simulink model "sfcndemo_frame"  (Simulink 7.6)
settings: Solver=FixedStepDiscrete  SolverMode=SingleTasking  StartTime=0.0  StopTime=1  RelTol=1e-3
PreLoadFcn:
  | a=ones(1,256);a(96:110)=zeros(1,15);a(148:162)=zeros(1,15);a=[a', a'];
Description:
  | (Requires Signal Processing Blockset) Frame-Based Processing for Removing Sinusoidal Noise Using C-MEX S-functions
settings Model: Creator=The MathWorks Inc.  ExtModeAutoUpdateStatusClock=off
settings OptimizationCC: BlockReduction=off  BooleanDataType=off  InitFltsAndDblsToZero=on
settings DebuggingCC: SaveWithParameterizedLinksMsg=none  SignalResolutionControl=TryResolveAllWithWarning  SolverPrmCheckMsg=none  MultiTaskDSMMsg=warning  MultiTaskCondExecSysMsg=none
settings HardwareCC: TargetUnknown=on
settings RTWCC: RetainRTWFile=on  IncludeERTFirstTime=on
settings CodeAppCC: CustomSymbolStrFcn=$F$N$M
settings GRTTargetCC: TargetFcnLib=ansi_tfl_tmw.mat

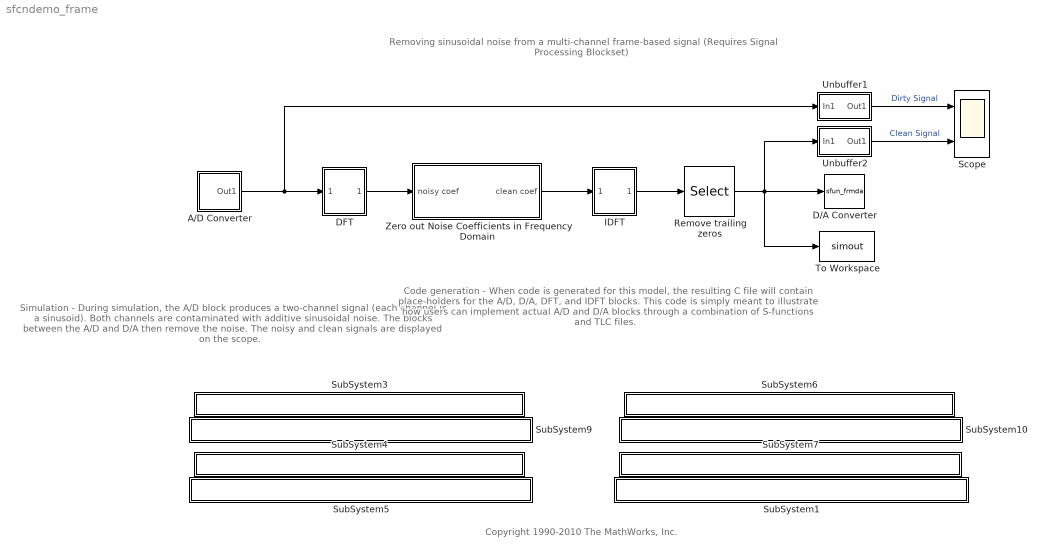
== system sfcndemo_frame ==
  note: Removing sinusoidal noise from a multi-channel frame-based signal
      | (Requires Signal Processing Blockset)
  note: Simulation -
      | During simulation, the A/D block produces
      | a two-channel signal (each channel is a sinusoid).
      | Both channels are contaminated with additive
      | sinusoidal noise. The blocks between the A/D and D/A
      | then remove the noise. The noisy and clean signals are
      | displayed on the scope.
  note: Code generation -
      | When code is generated for this model, the resulting C file
      | will contain place-holders for the A/D, D/A, DFT, and IDFT blocks.
      | This code is simply meant to illustrate how users can implement
      | actual A/D and D/A blocks through a combination of S-functions and
      | TLC files.
  note: Copyright 1990-2010 The MathWorks, Inc.
  A/D Converter : Subsystem  mask(A/D Converter){wf=Sine, amp=[10 5], freq=[5 10], Ts=0.005, fs=64, namp=4, nfreq=80}
      mask prompts: wf "Waveform for simulation"; amp "Amplitudes"; freq "Frequencies"; Ts "Sample time"; fs "Frame size"; namp "Noise amplitude for simulation"; nfreq "Noise frequency for simulation"
      mask help: During simulation, produces a constant or sinusoidal frame-based signal with additive sinusoidal noise. Multi-channel sinusoidal signals can be produced by giving a vector of frequncies or amplitudes. The same noise is added to all channels.
      mask StyleString: popup(Constant | Sine),edit,edit,edit,edit,edit,edit
      mask Display: disp('A/D')
  D/A Converter : S-Function  FunctionName=sfun_frmda  EnableBusSupport=off
      mask Type: D/A Converter
      mask Description: Frame-based D/A converter. Has no function during simulation.
      mask Display: disp('D/A')
  DFT : Subsystem  mask(DFT){ds=256}
      mask prompts: ds "DFT size"
      mask help: Compue the Discrete Fourer Transform
      mask Display: disp('DFT')
  IDFT : Subsystem
      mask Type: IDFT
      mask Description: Compute the inverse Discrete Fourier Transform.
      mask Display: disp('IDFT')
  Remove trailing zeros : Selector  NumberOfDimensions=2  IndexOptions=Index vector (dialog),Select all  Indices=1:64,-1  OutputSizes=1
  Scope : Scope  NumInputPorts=2
      settings: TimeRange=1  YMin=-12~-12  YMax=12~12
  SubSystem1 : Subsystem  mask{filename=sfun_frmunbuff.tlc}
      mask init:
      | x=sfundemo_maskdisp;
      settings: AttributesFormatString=\n  OpenFcn=sfundemo_openfcn
      mask Display: disp(x);
  SubSystem10 : Subsystem  mask{filename=sfun_frmdft.tlc}
      mask init:
      | x=sfundemo_maskdisp;
      settings: AttributesFormatString=\n  OpenFcn=sfundemo_openfcn
      mask Display: disp(x);
  SubSystem3 : Subsystem  mask{filename=sfun_frmad.c}
      mask init:
      | x=sfundemo_maskdisp;
      settings: AttributesFormatString=\n  OpenFcn=sfundemo_openfcn
      mask Display: disp(x);
  SubSystem4 : Subsystem  mask{filename=sfun_frmda.c}
      mask init:
      | x=sfundemo_maskdisp;
      settings: AttributesFormatString=\n  OpenFcn=sfundemo_openfcn
      mask Display: disp(x);
  SubSystem5 : Subsystem  mask{filename=sfun_frmda.tlc}
      mask init:
      | x=sfundemo_maskdisp;
      settings: AttributesFormatString=\n  OpenFcn=sfundemo_openfcn
      mask Display: disp(x);
  SubSystem6 : Subsystem  mask{filename=sfun_frmdft.c}
      mask init:
      | x=sfundemo_maskdisp;
      settings: AttributesFormatString=\n  OpenFcn=sfundemo_openfcn
      mask Display: disp(x);
  SubSystem7 : Subsystem  mask{filename=sfun_frmunbuff.c}
      mask init:
      | x=sfundemo_maskdisp;
      settings: AttributesFormatString=\n  OpenFcn=sfundemo_openfcn
      mask Display: disp(x);
  SubSystem9 : Subsystem  mask{filename=sfun_frmad.tlc}
      mask init:
      | x=sfundemo_maskdisp;
      settings: AttributesFormatString=\n  OpenFcn=sfundemo_openfcn
      mask Display: disp(x);
  To Workspace : ToWorkspace  VariableName=simout  SampleTime=-1  SaveFormat=Array
  Unbuffer1 : Subsystem
      mask Type: Frame Unbuffer
      mask Description: Unbuffer a frame-based signal
      mask Display: disp('Unbuffer')
  Unbuffer2 : Subsystem
      mask Type: Frame Unbuffer
      mask Description: Unbuffer a frame-based signal
      mask Display: disp('Unbuffer')
  Zero out Noise Coefficients in Frequency Domain : Subsystem
  wires:
  A/D Converter/1(Out1) -> DFT/1(In1), Unbuffer1/1(In1)
  DFT/1(Out1) -> Zero out Noise Coefficients in Frequency Domain/1(noisy coef)
  IDFT/1(Out1) -> Remove trailing zeros/1
  Remove trailing zeros/1 -> D/A Converter/1, Unbuffer2/1(In1), To Workspace/1
  Zero out Noise Coefficients in Frequency Domain/1(clean coef) -> IDFT/1(In1)
  Unbuffer2/1(Out1) -> Scope/2  "Clean Signal"
  Unbuffer1/1(Out1) -> Scope/1  "Dirty Signal"

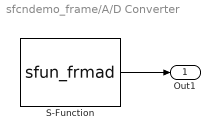
== system sfcndemo_frame/A/D Converter ==
  S-Function : S-Function  FunctionName=sfun_frmad  Parameters=wf,amp,freq,Ts,fs,namp,nfreq  SFunctionModules=sfun_frmad_wrapper  EnableBusSupport=off
  Out1 : Outport
  wires:
  S-Function/1 -> Out1/1

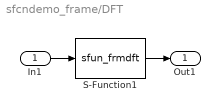
== system sfcndemo_frame/DFT ==
  In1 : Inport
  S-Function1 : S-Function  FunctionName=sfun_frmdft  Parameters=1,ds  SFunctionModules=sfun_frmdft_wrapper  EnableBusSupport=off
  Out1 : Outport
  wires:
  In1/1 -> S-Function1/1
  S-Function1/1 -> Out1/1

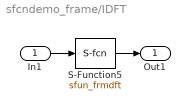
== system sfcndemo_frame/IDFT ==
  In1 : Inport
  S-Function5 : S-Function  FunctionName=sfun_frmdft  Parameters=2,256  SFunctionModules=sfun_frmdft_wrapper  EnableBusSupport=off
  Out1 : Outport
  wires:
  In1/1 -> S-Function5/1
  S-Function5/1 -> Out1/1

== system sfcndemo_frame/SubSystem1 ==

== system sfcndemo_frame/SubSystem10 ==

== system sfcndemo_frame/SubSystem3 ==

== system sfcndemo_frame/SubSystem4 ==

== system sfcndemo_frame/SubSystem5 ==

== system sfcndemo_frame/SubSystem6 ==

== system sfcndemo_frame/SubSystem7 ==

== system sfcndemo_frame/SubSystem9 ==

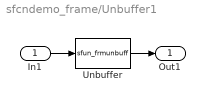
== system sfcndemo_frame/Unbuffer1 ==
  In1 : Inport
  Unbuffer : S-Function  FunctionName=sfun_frmunbuff  SFunctionModules=sfun_frmunbuff_wrapper  EnableBusSupport=off
  Out1 : Outport
  wires:
  Unbuffer/1 -> Out1/1
  In1/1 -> Unbuffer/1

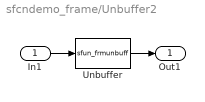
== system sfcndemo_frame/Unbuffer2 ==
  In1 : Inport
  Unbuffer : S-Function  FunctionName=sfun_frmunbuff  SFunctionModules=sfun_frmunbuff_wrapper  EnableBusSupport=off
  Out1 : Outport
  wires:
  In1/1 -> Unbuffer/1
  Unbuffer/1 -> Out1/1

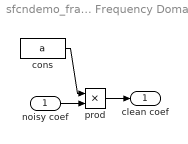
== system sfcndemo_frame/Zero out Noise Coefficients in Frequency Domain ==
  noisy coef : Inport
  cons : Constant  Value=a
  prod : Product  SaturateOnIntegerOverflow=on  InputSameDT=on  OutDataTypeStr=Inherit: Same as first input
  clean coef : Outport
  wires:
  cons/1 -> prod/1
  prod/1 -> clean coef/1
  noisy coef/1 -> prod/2
